simulink model "SimulinkOminidirectinalDrone_restored_from_autosave"  (R2025a)
settings: Solver=ode15s  StartTime=0.0  StopTime=10  RelTol=1e-4
values from neighbouring files (symbols this model uses):
  AUM = 3.057    [Parameter.m]
  g = -9.8    [Parameter.m]
  H = 0.05    [Parameter.m]
  L = 0.25    [Parameter.m]
  rho = 1.18195    [Parameter.m]
  W = diag([0.994, 0.003, 0.003, 0.994, 0.003, 0.003,            0.994, 0.003, 0.003, 0.994, 0.003, 0.003])    [Parameter.m]
libraries: slpidlib x10, matrix_library x8, robotcorelib x4, simulink x1, uavalgslib x1, aerolibobsolete x1
(part 1 of 2)
settings Model: Creator=Nguyen_Duc  LastModifiedBy=Nguyen_Duc
settings RTWCC: GPUComputeCapability=3.5

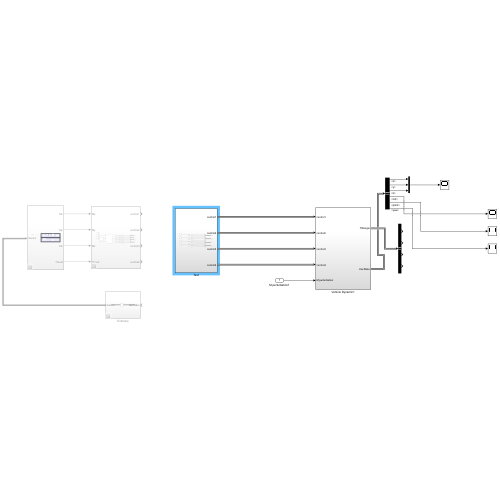
[thumbnail: Simulink's stored preview of the top-level diagram]
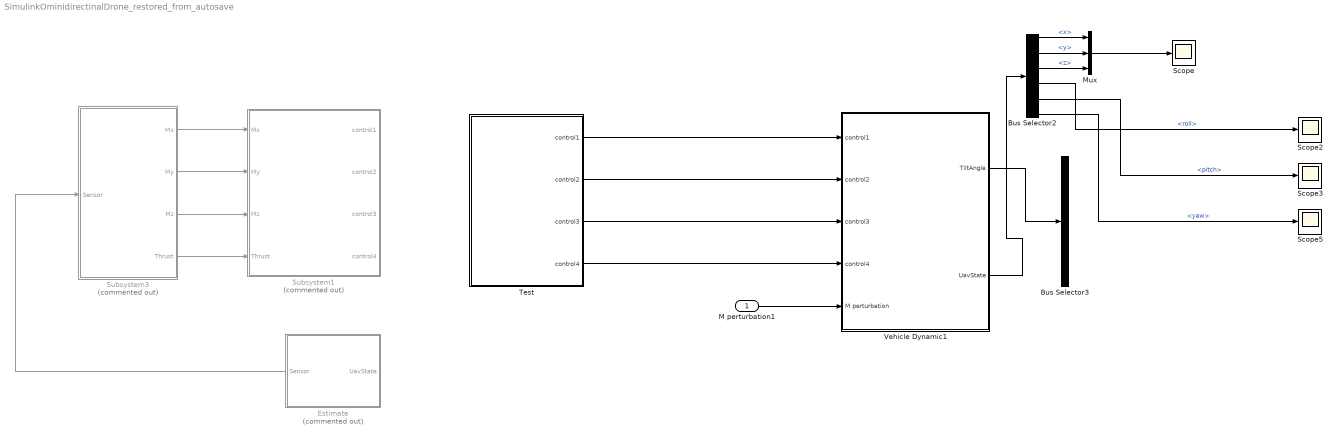
== system SimulinkOminidirectinalDrone_restored_from_autosave ==
  M perturbation1 : Inport
  Bus Selector2 : BusSelector  OutputSignals=x,y,z,roll,pitch,yaw
  Bus Selector3 : BusSelector  OutputSignals=signal1,signal2,signal3,signal4
  Estimate : Subsystem  Commented=on
  Mux : Mux  Inputs=3
  Scope{,2..3,5} (4 alike) : Scope
      Scope settings: ActiveDisplayYMinimum=-3203.8909963657634  ActiveDisplayYMaximum=3110.7651508209105
      Scope2 settings: ActiveDisplayYMinimum=-2.0964114847916129  ActiveDisplayYMaximum=2.211139771042796  DataLoggingVariableName=ScopeData2
      Scope3 settings: ActiveDisplayYMinimum=-3.8093227520417652  ActiveDisplayYMaximum=3.6702175311661223  DataLoggingVariableName=ScopeData3
      Scope5 settings: ActiveDisplayYMinimum=-9.534765072380404  ActiveDisplayYMaximum=7.24447859071625  DataLoggingVariableName=ScopeData5
  Subsystem1 : Subsystem  Commented=on
  Subsystem3 : Subsystem  Commented=on
  Test : Subsystem
  Vehicle Dynamic1 : Subsystem
  wires:
  Bus Selector2/1 -> Mux/1  "<x>"
  Subsystem3/3(Mz) -> Subsystem1/3(Mz)
  Subsystem3/1(Mx) -> Subsystem1/1(Mx)
  Bus Selector2/5 -> Scope3/1  "<pitch>"
  Subsystem3/2(My) -> Subsystem1/2(My)
  M perturbation1/1 -> Vehicle Dynamic1/5(M perturbation)
  Vehicle Dynamic1/1(TiltAngle) -> Bus Selector3/1
  Bus Selector2/6 -> Scope5/1  "<yaw>"
  Bus Selector2/3 -> Mux/3  "<z>"
  Subsystem3/4(Thrust) -> Subsystem1/4(Thrust)
  Bus Selector2/4 -> Scope2/1  "<roll>"
  Bus Selector2/2 -> Mux/2  "<y>"
  Vehicle Dynamic1/2(UavState) -> Bus Selector2/1
  Mux/1 -> Scope/1
  Estimate/1(Sensor) -> Subsystem3/1(Sensor)
  Test/1(control1) -> Vehicle Dynamic1/1(control1)
  Test/2(control2) -> Vehicle Dynamic1/2(control2)
  Test/3(control3) -> Vehicle Dynamic1/3(control3)
  Test/4(control4) -> Vehicle Dynamic1/4(control4)

== system SimulinkOminidirectinalDrone_restored_from_autosave/Estimate ==
  UavState : Inport
  Rate Transition : RateTransition  OutPortSampleTime=0.005
  Sensor : Outport
  wires:
  UavState/1 -> Rate Transition/1
  Rate Transition/1 -> Sensor/1

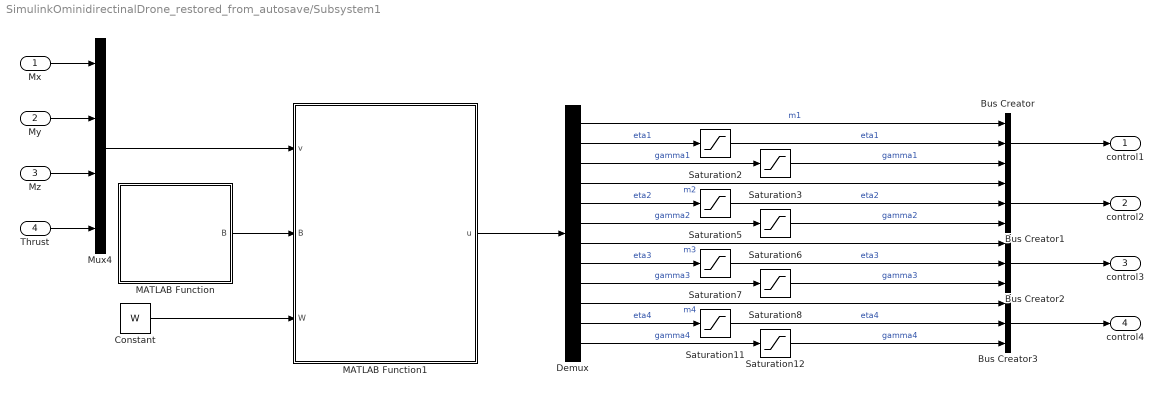
== system SimulinkOminidirectinalDrone_restored_from_autosave/Subsystem1 ==
  Mx : Inport
  My : Inport  Port=2
  Mz : Inport  Port=3
  Thrust : Inport  Port=4
  Bus Creator{,1..3} (4 alike) : BusCreator  Inputs=3
  Constant : Constant  Value=W
  Demux : Demux  Outputs=12
  MATLAB Function : MATLAB Function  TreatAsAtomicUnit=on
  MATLAB Function1 : MATLAB Function  TreatAsAtomicUnit=on
  Mux4 : Mux
  Saturation{2..3,5..8,11..12} (8 alike) : Saturate  UpperLimit=20*pi/180  LowerLimit=-20*pi/180
  control1 : Outport
  control2 : Outport  Port=2
  control3 : Outport  Port=3
  control4 : Outport  Port=4
  wires:
  MATLAB Function/1(B) -> MATLAB Function1/2(B)
  Mux4/1 -> MATLAB Function1/1(v)
  Demux/1 -> Bus Creator/1  "m1"
  Bus Creator/1 -> control1/1
  Demux/3 -> Saturation3/1  "gamma1"
  Demux/2 -> Saturation2/1  "eta1"
  Demux/4 -> Bus Creator1/1  "m2"
  Demux/5 -> Saturation5/1  "eta2"
  Demux/6 -> Saturation6/1  "gamma2"
  Demux/7 -> Bus Creator2/1  "m3"
  Demux/8 -> Saturation7/1  "eta3"
  Demux/9 -> Saturation8/1  "gamma3"
  Demux/10 -> Bus Creator3/1  "m4"
  Demux/11 -> Saturation11/1  "eta4"
  Demux/12 -> Saturation12/1  "gamma4"
  Bus Creator1/1 -> control2/1
  Bus Creator2/1 -> control3/1
  Bus Creator3/1 -> control4/1
  Mx/1 -> Mux4/1
  My/1 -> Mux4/2
  Mz/1 -> Mux4/3
  Thrust/1 -> Mux4/4
  Constant/1 -> MATLAB Function1/3(W)
  MATLAB Function1/1(u) -> Demux/1
  Saturation2/1 -> Bus Creator/2  "eta1"
  Saturation3/1 -> Bus Creator/3  "gamma1"
  Saturation5/1 -> Bus Creator1/2  "eta2"
  Saturation6/1 -> Bus Creator1/3  "gamma2"
  Saturation7/1 -> Bus Creator2/2  "eta3"
  Saturation8/1 -> Bus Creator2/3  "gamma3"
  Saturation11/1 -> Bus Creator3/2  "eta4"
  Saturation12/1 -> Bus Creator3/3  "gamma4"

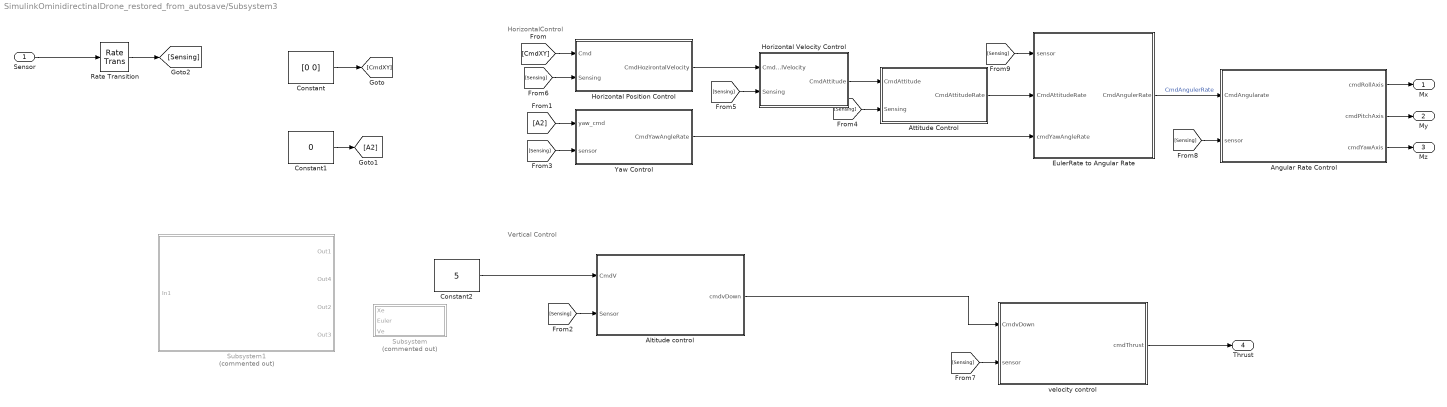
== system SimulinkOminidirectinalDrone_restored_from_autosave/Subsystem3 ==
  note: HorizontalControl
  note: Vertical Control
  Sensor : Inport
  Altitude control : Subsystem
  Angular Rate Control : Subsystem
  Attitude Control : Subsystem
  Constant : Constant  Value=[0 0]
  Constant1 : Constant  Value=0
  Constant2 : Constant  Value=5
  EulerRate to Angular Rate : Subsystem
  Horizontal Position Control : Subsystem
  Horizontal Velocity Control : Subsystem
  Rate Transition : RateTransition  OutPortSampleTime=0.005
  Subsystem : Subsystem  Commented=on
  Subsystem1 : Subsystem  Commented=on
  Yaw Control : Subsystem
  velocity control : Subsystem
  Mx : Outport
  My : Outport  Port=2
  Mz : Outport  Port=3
  Thrust : Outport  Port=4
  wires:
  Sensor/1 -> Rate Transition/1
  velocity control/1(cmdThrust) -> Thrust/1
  Altitude control/1(cmdvDown) -> velocity control/1(CmdvDown)
  EulerRate to Angular Rate/1(CmdAngulerRate) -> Angular Rate Control/1(CmdAngularate)  "CmdAngulerRate"
  Attitude Control/1(CmdAttitudeRate) -> EulerRate to Angular Rate/2(CmdAttitudeRate)
  Horizontal Velocity Control/1(CmdAttitude) -> Attitude Control/1(CmdAttitude)
  Horizontal Position Control/1(CmdHozirontalVelocity) -> Horizontal Velocity Control/1(CmdHozirontalVelocity)
  Yaw Control/1(CmdYawAngleRate) -> EulerRate to Angular Rate/3(cmdYawAngleRate)
  Angular Rate Control/1(cmdRollAxis) -> Mx/1
  Angular Rate Control/3(cmdYawAxis) -> Mz/1
  Angular Rate Control/2(cmdPitchAxis) -> My/1
  Constant/1 -> [CmdXY]
  [CmdXY] -> Horizontal Position Control/1(Cmd)
  Constant1/1 -> [A2]
  [A2] -> Yaw Control/1(yaw_cmd)
  Constant2/1 -> Altitude control/1(CmdV)
  Rate Transition/1 -> [Sensing]
  [Sensing] -> Altitude control/2(Sensor)
  [Sensing] -> Yaw Control/2(sensor)
  [Sensing] -> Attitude Control/2(Sensing)
  [Sensing] -> Horizontal Velocity Control/2(Sensing)
  [Sensing] -> Horizontal Position Control/2(Sensing)
  [Sensing] -> velocity control/2(sensor)
  [Sensing] -> Angular Rate Control/2(sensor)
  [Sensing] -> EulerRate to Angular Rate/1(sensor)

== system SimulinkOminidirectinalDrone_restored_from_autosave/Test ==
  Bus Creator{,1..3} (4 alike) : BusCreator  Inputs=3
  Constant : Constant  Value=2000
  Constant{1..2,4..5,7..8,10..11} (8 alike) : Constant
  Constant3 : Constant  Value=2000
  Constant6 : Constant  Value=1000
  Constant9 : Constant  Value=2000
  control1 : Outport
  control2 : Outport  Port=2
  control3 : Outport  Port=3
  control4 : Outport  Port=4
  wires:
  Constant1/1 -> Bus Creator/2  "eta1"
  Bus Creator1/1 -> control2/1
  Constant4/1 -> Bus Creator1/2  "eta2"
  Constant5/1 -> Bus Creator1/3  "gamma2"
  Bus Creator2/1 -> control3/1
  Constant3/1 -> Bus Creator1/1  "m2"
  Constant10/1 -> Bus Creator3/2  "eta4"
  Constant2/1 -> Bus Creator/3  "gamma1"
  Bus Creator/1 -> control1/1
  Constant7/1 -> Bus Creator2/2  "eta3"
  Constant11/1 -> Bus Creator3/3  "gamma4"
  Constant8/1 -> Bus Creator2/3  "gamma3"
  Bus Creator3/1 -> control4/1
  Constant6/1 -> Bus Creator2/1  "m3"
  Constant/1 -> Bus Creator/1  "m1"
  Constant9/1 -> Bus Creator3/1  "m4"

== system SimulinkOminidirectinalDrone_restored_from_autosave/Vehicle Dynamic1 ==
  control1 : Inport
  control2 : Inport  Port=2
  control3 : Inport  Port=3
  control4 : Inport  Port=4
  M perturbation : Inport  Port=5
  6DOF (Euler Angles) : aerolibobsolete/6DOF (Euler Angles)  units=Metric (MKS)  mtype=Fixed  rep=Euler Angles  xme_0=[0 0 0]  Vm_0=[0 0 0]  eul_0=[0 0 0]  pm_0=[0 0 0]  mass_0=AUM  mass_e=0.5  mass_f=2.0  inertia=[0.049827 0 0; 0 0.048993 0; 0 0 0.082777]  inertia_e=eye(3)  inertia_f=2*eye(3)  k_quat=1.0  vre_flag=on  abi_flag=off  aMode=0  xme_statename=''  Vm_statename=''  eul_statename=''  quat_statename=''  pm_statename=''  mass_statename=''
  Constant : Constant  Value=[0 0 g*AUM]'
  Matrix Multiply : Product  Multiplication=Matrix(*)
  Subsystem1 : Subsystem
  Sum : Sum  Inputs=++|
  Sum1 : Sum  Inputs=|++
  Uav : Subsystem
  actuator : Subsystem
  TiltAngle : Outport
  UavState : Outport  Port=2
  wires:
  control3/1 -> actuator/4(control3)
  M perturbation/1 -> Sum1/2
  Matrix Multiply/1 -> Sum/1
  control1/1 -> actuator/2(control1)
  control2/1 -> actuator/3(control2)
  control4/1 -> actuator/5(control4)
  Constant/1 -> Matrix Multiply/2
  6DOF (Euler Angles)/6 -> Uav/6(pqr), Subsystem1/1(omega)  "pqr"
  6DOF (Euler Angles)/5 -> Uav/5(vb), actuator/6(Vb)  "vb"
  6DOF (Euler Angles)/4 -> Uav/4(dcm), Matrix Multiply/1  "dcm"
  actuator/3(TiltAngle) -> TiltAngle/1
  Subsystem1/1(Rotation) -> actuator/1(rotation)
  Sum/1 -> 6DOF (Euler Angles)/1
  actuator/1(Forces) -> Sum/2
  actuator/2(Moments) -> Sum1/1
  Sum1/1 -> 6DOF (Euler Angles)/2
  6DOF (Euler Angles)/1 -> Uav/1(ve)  "ve"
  6DOF (Euler Angles)/2 -> Uav/2(xe)  "xe"
  6DOF (Euler Angles)/3 -> Uav/3(euler)  "euler"
  6DOF (Euler Angles)/7 -> Uav/7(angular acce)  "angular acce"
  6DOF (Euler Angles)/8 -> Uav/8(accel)  "accel"
  Uav/1(UavState) -> UavState/1

== system SimulinkOminidirectinalDrone_restored_from_autosave/Subsystem3/Altitude control ==
  CmdV : Inport
  In Bus Element1 : Inport  Port=2  PortName=Sensor  Element=z
  Discrete PID Controller : slpidlib/PID Controller  Controller=PD  Form=Parallel  TimeDomain=Discrete-time  UseExternalTs=off  SampleTime=0.005  IntegratorMethod=Forward Euler  FilterMethod=Forward Euler  ControllerParametersSource=internal  P=100  I=1  UseKiTs=off  D=1000  UseExternalDerivativeSource=off  N=100  UseFilter=on  TunerSelectOption=Transfer Function Based (PID Tuner App)  InitialConditionSource=external  InitialConditionForIntegrator=0  InitialConditionForFilter=0  DifferentiatorICPrevScaledInput=0  ExternalReset=none  TrackingMode=off  Kt=1  LimitOutput=on  SatLimitsSource=internal  UpperSaturationLimit=inf  LowerSaturationLimit=-inf  LinearizeAsGain=off  AntiWindupMode=none  Kb=1  LimitIntegrator=off  UpperIntegratorSaturationLimit=inf  LowerIntegratorSaturationLimit=-inf  POutMin=[]  POutMax=[]  IOutMin=[]  IOutMax=[]  DOutMin=[]  DOutMax=[]  NOutMin=[]  NOutMax=[]  SumOutMin=[]  SumOutMax=[]  SaturationOutMin=[]  SaturationOutMax=[]  PParamMin=[]  PParamMax=[]  IParamMin=[]  IParamMax=[]  DParamMin=[]  DParamMax=[]  NParamMin=[]  NParamMax=[]  KbParamMin=[]  KbParamMax=[]  KtParamMin=[]  KtParamMax=[]  KbOutMin=[]  KbOutMax=[]  KtOutMin=[]  KtOutMax=[]  IntegratorOutMin=[]  IntegratorOutMax=[]  FilterOutMin=[]  FilterOutMax=[]  SumI1OutMin=[]  SumI1OutMax=[]  SumI2OutMin=[]  SumI2OutMax=[]  SumI3OutMin=[]  SumI3OutMax=[]  SumI4OutMin=[]  SumI4OutMax=[]  SumDOutMin=[]  SumDOutMax=[]  DifferentiatorOutMin=[]  DifferentiatorOutMax=[]  FilterDiffOutCoefMin=[]  FilterDiffOutCoefMax=[]  ReciprocalOutMin=[]  ReciprocalOutMax=[]  SumDenOutMin=[]  SumDenOutMax=[]  SumNumOutMin=[]  SumNumOutMax=[]  DivideOutMin=[]  DivideOutMax=[]  UdiffTsProdOutMin=[]  UdiffTsProdOutMax=[]  NTsProdOutMin=[]  NTsProdOutMax=[]  UintegralTsProdOutMin=[]  UintegralTsProdOutMax=[]  UngainTsProdOutMin=[]  UngainTsProdOutMax=[]  ClampingZeroOutDataTypeStr=Inherit: Inherit via back propagation  ClampingZeroOutMin=[]  ClampingZeroOutMax=[]  FilterDenConstantOutDataTypeStr=Inherit: Inherit via back propagation  FilterDenConstantOutMin=[]  FilterDenConstantOutMax=[]  PCopyOutDataTypeStr=Inherit: Inherit via back propagation  PCopyOutMin=[]  PCopyOutMax=[]  NCopyOutDataTypeStr=Inherit: Inherit via back propagation  NCopyOutMin=[]  NCopyOutMax=[]  IntegratorContinuousStateAttributes=''  IntegratorStateMustResolveToSignalObject=off  IntegratorRTWStateStorageClass=Auto  FilterContinuousStateAttributes=''  FilterStateMustResolveToSignalObject=off  FilterRTWStateStorageClass=Auto  ParallelPVariant=InternalParameters  IdealPVariant=Disabled  IVariant=Disabled  DVariant=InternalParameters  IntegratorVariant=Disabled  SatVariant=Enabled  AWVariant=Disabled  PCopyVariant=Disabled  TRVariant=Disabled  FdbkBlocksVariant=Forward  IdealPFdbkVariant=Disabled  SatFdbkVariant=Disabled  DerivativeFilterVariant=ForwardEulerFilter  NVariant=InternalParameters  NCopyVariant=Disabled  FilterICVariant=ExternalICs  IntegratorICVariant=Disabled  ExternalResetVariant=Disabled  TRSumVariant=Passthrough  SumFdbkVariant=Disabled  SumVariant=Sum_PD  TsampFilterVariant=InternalTs  TsampNgainVariant=Passthrough  TsampIntegralVariant=Disabled_SignalSpec  ExternalSaturationOutDataTypeStr=Inherit: Same as second input  DerivativeSourceVariant=ErrorSignal  PreIntVariant=InternalPreInt
      settings: LibrarySourceBlock=simulink/Discrete/Discrete PID Controller
  Gain : Gain  Gain=-2
  Sum : Sum  Inputs=|+-
  cmdvDown : Outport
  wires:
  Sum/1 -> Discrete PID Controller/1
  In Bus Element1/1 -> Sum/2
  CmdV/1 -> Gain/1
  Discrete PID Controller/1 -> cmdvDown/1  "cmdvDown"
  Gain/1 -> Sum/1

== system SimulinkOminidirectinalDrone_restored_from_autosave/Subsystem3/Angular Rate Control ==
  In Bus Element : Inport  PortName=CmdAngularate  Element=wx
  In Bus Element1 : Inport  PortName=CmdAngularate  Element=wy
  In Bus Element4 : Inport  PortName=CmdAngularate  Element=wz
  In Bus Element2 : Inport  Port=2  PortName=sensor  Element=wy
  In Bus Element3 : Inport  Port=2  PortName=sensor  Element=wx
  In Bus Element5 : Inport  Port=2  PortName=sensor  Element=wz
  Demux : Demux  Outputs=2
  Discrete PID Controller : slpidlib/PID Controller  Controller=PID  Form=Parallel  TimeDomain=Discrete-time  UseExternalTs=off  SampleTime=-1  IntegratorMethod=Forward Euler  FilterMethod=Forward Euler  ControllerParametersSource=internal  P=1  I=0  UseKiTs=off  D=0  UseExternalDerivativeSource=off  N=100  UseFilter=on  TunerSelectOption=Transfer Function Based (PID Tuner App)  InitialConditionSource=internal  InitialConditionForIntegrator=0  InitialConditionForFilter=0  DifferentiatorICPrevScaledInput=0  ExternalReset=none  TrackingMode=off  Kt=1  LimitOutput=off  SatLimitsSource=internal  UpperSaturationLimit=inf  LowerSaturationLimit=-inf  LinearizeAsGain=off  AntiWindupMode=none  Kb=1  LimitIntegrator=off  UpperIntegratorSaturationLimit=inf  LowerIntegratorSaturationLimit=-inf  POutMin=[]  POutMax=[]  IOutMin=[]  IOutMax=[]  DOutMin=[]  DOutMax=[]  NOutMin=[]  NOutMax=[]  SumOutMin=[]  SumOutMax=[]  SaturationOutMin=[]  SaturationOutMax=[]  PParamMin=[]  PParamMax=[]  IParamMin=[]  IParamMax=[]  DParamMin=[]  DParamMax=[]  NParamMin=[]  NParamMax=[]  KbParamMin=[]  KbParamMax=[]  KtParamMin=[]  KtParamMax=[]  KbOutMin=[]  KbOutMax=[]  KtOutMin=[]  KtOutMax=[]  IntegratorOutMin=[]  IntegratorOutMax=[]  FilterOutMin=[]  FilterOutMax=[]  SumI1OutMin=[]  SumI1OutMax=[]  SumI2OutMin=[]  SumI2OutMax=[]  SumI3OutMin=[]  SumI3OutMax=[]  SumI4OutMin=[]  SumI4OutMax=[]  SumDOutMin=[]  SumDOutMax=[]  DifferentiatorOutMin=[]  DifferentiatorOutMax=[]  FilterDiffOutCoefMin=[]  FilterDiffOutCoefMax=[]  ReciprocalOutMin=[]  ReciprocalOutMax=[]  SumDenOutMin=[]  SumDenOutMax=[]  SumNumOutMin=[]  SumNumOutMax=[]  DivideOutMin=[]  DivideOutMax=[]  UdiffTsProdOutMin=[]  UdiffTsProdOutMax=[]  NTsProdOutMin=[]  NTsProdOutMax=[]  UintegralTsProdOutMin=[]  UintegralTsProdOutMax=[]  UngainTsProdOutMin=[]  UngainTsProdOutMax=[]  ClampingZeroOutDataTypeStr=Inherit: Inherit via back propagation  ClampingZeroOutMin=[]  ClampingZeroOutMax=[]  FilterDenConstantOutDataTypeStr=Inherit: Inherit via back propagation  FilterDenConstantOutMin=[]  FilterDenConstantOutMax=[]  PCopyOutDataTypeStr=Inherit: Inherit via back propagation  PCopyOutMin=[]  PCopyOutMax=[]  NCopyOutDataTypeStr=Inherit: Inherit via back propagation  NCopyOutMin=[]  NCopyOutMax=[]  IntegratorContinuousStateAttributes=''  IntegratorStateMustResolveToSignalObject=off  IntegratorRTWStateStorageClass=Auto  FilterContinuousStateAttributes=''  FilterStateMustResolveToSignalObject=off  FilterRTWStateStorageClass=Auto  ParallelPVariant=InternalParameters  IdealPVariant=Disabled  IVariant=InternalParameters  DVariant=InternalParameters  IntegratorVariant=Discrete  SatVariant=Disabled  AWVariant=Passthrough  PCopyVariant=Disabled  TRVariant=Disabled  FdbkBlocksVariant=Forward  IdealPFdbkVariant=Disabled  SatFdbkVariant=Disabled  DerivativeFilterVariant=ForwardEulerFilter  NVariant=InternalParameters  NCopyVariant=Disabled  FilterICVariant=InternalICsFilter  IntegratorICVariant=InternalICs  ExternalResetVariant=Disabled  TRSumVariant=Passthrough  SumFdbkVariant=Disabled  SumVariant=Sum_PID  TsampFilterVariant=InternalTs  TsampNgainVariant=Passthrough  TsampIntegralVariant=Disabled_SignalSpec  ExternalSaturationOutDataTypeStr=Inherit: Same as second input  DerivativeSourceVariant=ErrorSignal  PreIntVariant=InternalPreInt
      settings: LibrarySourceBlock=simulink/Discrete/Discrete PID Controller
  Discrete PID Controller1 : slpidlib/PID Controller  Controller=PID  Form=Parallel  TimeDomain=Discrete-time  UseExternalTs=off  SampleTime=-1  IntegratorMethod=Forward Euler  FilterMethod=Forward Euler  ControllerParametersSource=internal  P=1  I=0  UseKiTs=off  D=0  UseExternalDerivativeSource=off  N=100  UseFilter=on  TunerSelectOption=Transfer Function Based (PID Tuner App)  InitialConditionSource=internal  InitialConditionForIntegrator=0  InitialConditionForFilter=0  DifferentiatorICPrevScaledInput=0  ExternalReset=none  TrackingMode=off  Kt=1  LimitOutput=off  SatLimitsSource=internal  UpperSaturationLimit=inf  LowerSaturationLimit=-inf  LinearizeAsGain=off  AntiWindupMode=none  Kb=1  LimitIntegrator=off  UpperIntegratorSaturationLimit=inf  LowerIntegratorSaturationLimit=-inf  POutMin=[]  POutMax=[]  IOutMin=[]  IOutMax=[]  DOutMin=[]  DOutMax=[]  NOutMin=[]  NOutMax=[]  SumOutMin=[]  SumOutMax=[]  SaturationOutMin=[]  SaturationOutMax=[]  PParamMin=[]  PParamMax=[]  IParamMin=[]  IParamMax=[]  DParamMin=[]  DParamMax=[]  NParamMin=[]  NParamMax=[]  KbParamMin=[]  KbParamMax=[]  KtParamMin=[]  KtParamMax=[]  KbOutMin=[]  KbOutMax=[]  KtOutMin=[]  KtOutMax=[]  IntegratorOutMin=[]  IntegratorOutMax=[]  FilterOutMin=[]  FilterOutMax=[]  SumI1OutMin=[]  SumI1OutMax=[]  SumI2OutMin=[]  SumI2OutMax=[]  SumI3OutMin=[]  SumI3OutMax=[]  SumI4OutMin=[]  SumI4OutMax=[]  SumDOutMin=[]  SumDOutMax=[]  DifferentiatorOutMin=[]  DifferentiatorOutMax=[]  FilterDiffOutCoefMin=[]  FilterDiffOutCoefMax=[]  ReciprocalOutMin=[]  ReciprocalOutMax=[]  SumDenOutMin=[]  SumDenOutMax=[]  SumNumOutMin=[]  SumNumOutMax=[]  DivideOutMin=[]  DivideOutMax=[]  UdiffTsProdOutMin=[]  UdiffTsProdOutMax=[]  NTsProdOutMin=[]  NTsProdOutMax=[]  UintegralTsProdOutMin=[]  UintegralTsProdOutMax=[]  UngainTsProdOutMin=[]  UngainTsProdOutMax=[]  ClampingZeroOutDataTypeStr=Inherit: Inherit via back propagation  ClampingZeroOutMin=[]  ClampingZeroOutMax=[]  FilterDenConstantOutDataTypeStr=Inherit: Inherit via back propagation  FilterDenConstantOutMin=[]  FilterDenConstantOutMax=[]  PCopyOutDataTypeStr=Inherit: Inherit via back propagation  PCopyOutMin=[]  PCopyOutMax=[]  NCopyOutDataTypeStr=Inherit: Inherit via back propagation  NCopyOutMin=[]  NCopyOutMax=[]  IntegratorContinuousStateAttributes=''  IntegratorStateMustResolveToSignalObject=off  IntegratorRTWStateStorageClass=Auto  FilterContinuousStateAttributes=''  FilterStateMustResolveToSignalObject=off  FilterRTWStateStorageClass=Auto  ParallelPVariant=InternalParameters  IdealPVariant=Disabled  IVariant=InternalParameters  DVariant=InternalParameters  IntegratorVariant=Discrete  SatVariant=Disabled  AWVariant=Passthrough  PCopyVariant=Disabled  TRVariant=Disabled  FdbkBlocksVariant=Forward  IdealPFdbkVariant=Disabled  SatFdbkVariant=Disabled  DerivativeFilterVariant=ForwardEulerFilter  NVariant=InternalParameters  NCopyVariant=Disabled  FilterICVariant=InternalICsFilter  IntegratorICVariant=InternalICs  ExternalResetVariant=Disabled  TRSumVariant=Passthrough  SumFdbkVariant=Disabled  SumVariant=Sum_PID  TsampFilterVariant=InternalTs  TsampNgainVariant=Passthrough  TsampIntegralVariant=Disabled_SignalSpec  ExternalSaturationOutDataTypeStr=Inherit: Same as second input  DerivativeSourceVariant=ErrorSignal  PreIntVariant=InternalPreInt
      settings: LibrarySourceBlock=simulink/Discrete/Discrete PID Controller
  Gain : Gain  Gain=20
  Gain1 : Gain  Gain=100
  Mux : Mux  Inputs=2
  Mux1 : Mux  Inputs=2
  Sum : Sum  Inputs=|+-
  Sum1 : Sum  Inputs=|+-
  cmdRollAxis : Outport
  cmdPitchAxis : Outport  Port=2
  cmdYawAxis : Outport  Port=3
  wires:
  In Bus Element/1 -> Mux/1
  In Bus Element1/1 -> Mux/2
  In Bus Element3/1 -> Mux1/1
  In Bus Element2/1 -> Mux1/2
  Mux/1 -> Sum/1
  Mux1/1 -> Sum/2
  Sum/1 -> Discrete PID Controller/1
  Discrete PID Controller/1 -> Gain/1
  Gain/1 -> Demux/1
  Demux/2 -> cmdPitchAxis/1
  Demux/1 -> cmdRollAxis/1
  In Bus Element4/1 -> Sum1/1
  In Bus Element5/1 -> Sum1/2
  Sum1/1 -> Discrete PID Controller1/1
  Discrete PID Controller1/1 -> Gain1/1
  Gain1/1 -> cmdYawAxis/1

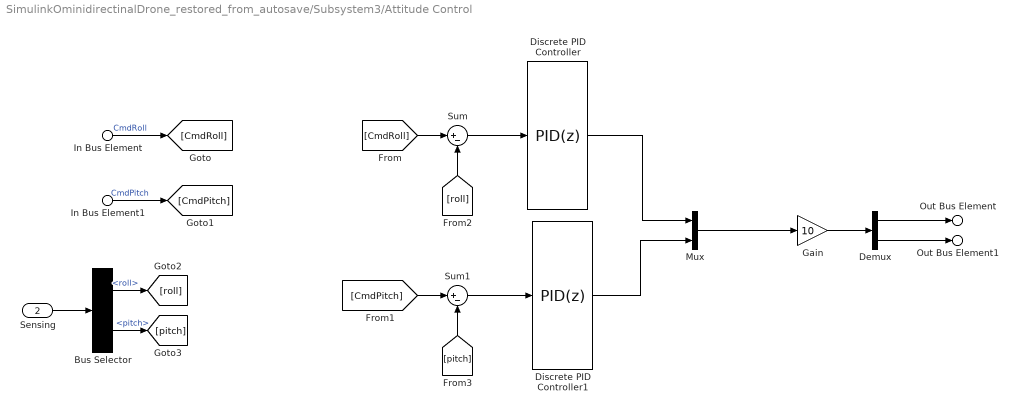
== system SimulinkOminidirectinalDrone_restored_from_autosave/Subsystem3/Attitude Control ==
  In Bus Element : Inport  PortName=CmdAttitude  Element=roll
  In Bus Element1 : Inport  PortName=CmdAttitude  Element=pitch
  Sensing : Inport  Port=2
  Bus Selector : BusSelector  OutputSignals=roll,pitch
  Demux : Demux  Outputs=2
  Discrete PID Controller : slpidlib/PID Controller  Controller=PID  Form=Parallel  TimeDomain=Discrete-time  UseExternalTs=off  SampleTime=-1  IntegratorMethod=Forward Euler  FilterMethod=Forward Euler  ControllerParametersSource=internal  P=1  I=0  UseKiTs=off  D=0  UseExternalDerivativeSource=off  N=100  UseFilter=on  TunerSelectOption=Transfer Function Based (PID Tuner App)  InitialConditionSource=internal  InitialConditionForIntegrator=0  InitialConditionForFilter=0  DifferentiatorICPrevScaledInput=0  ExternalReset=none  TrackingMode=off  Kt=1  LimitOutput=off  SatLimitsSource=internal  UpperSaturationLimit=inf  LowerSaturationLimit=-inf  LinearizeAsGain=off  AntiWindupMode=none  Kb=1  LimitIntegrator=off  UpperIntegratorSaturationLimit=inf  LowerIntegratorSaturationLimit=-inf  POutMin=[]  POutMax=[]  IOutMin=[]  IOutMax=[]  DOutMin=[]  DOutMax=[]  NOutMin=[]  NOutMax=[]  SumOutMin=[]  SumOutMax=[]  SaturationOutMin=[]  SaturationOutMax=[]  PParamMin=[]  PParamMax=[]  IParamMin=[]  IParamMax=[]  DParamMin=[]  DParamMax=[]  NParamMin=[]  NParamMax=[]  KbParamMin=[]  KbParamMax=[]  KtParamMin=[]  KtParamMax=[]  KbOutMin=[]  KbOutMax=[]  KtOutMin=[]  KtOutMax=[]  IntegratorOutMin=[]  IntegratorOutMax=[]  FilterOutMin=[]  FilterOutMax=[]  SumI1OutMin=[]  SumI1OutMax=[]  SumI2OutMin=[]  SumI2OutMax=[]  SumI3OutMin=[]  SumI3OutMax=[]  SumI4OutMin=[]  SumI4OutMax=[]  SumDOutMin=[]  SumDOutMax=[]  DifferentiatorOutMin=[]  DifferentiatorOutMax=[]  FilterDiffOutCoefMin=[]  FilterDiffOutCoefMax=[]  ReciprocalOutMin=[]  ReciprocalOutMax=[]  SumDenOutMin=[]  SumDenOutMax=[]  SumNumOutMin=[]  SumNumOutMax=[]  DivideOutMin=[]  DivideOutMax=[]  UdiffTsProdOutMin=[]  UdiffTsProdOutMax=[]  NTsProdOutMin=[]  NTsProdOutMax=[]  UintegralTsProdOutMin=[]  UintegralTsProdOutMax=[]  UngainTsProdOutMin=[]  UngainTsProdOutMax=[]  ClampingZeroOutDataTypeStr=Inherit: Inherit via back propagation  ClampingZeroOutMin=[]  ClampingZeroOutMax=[]  FilterDenConstantOutDataTypeStr=Inherit: Inherit via back propagation  FilterDenConstantOutMin=[]  FilterDenConstantOutMax=[]  PCopyOutDataTypeStr=Inherit: Inherit via back propagation  PCopyOutMin=[]  PCopyOutMax=[]  NCopyOutDataTypeStr=Inherit: Inherit via back propagation  NCopyOutMin=[]  NCopyOutMax=[]  IntegratorContinuousStateAttributes=''  IntegratorStateMustResolveToSignalObject=off  IntegratorRTWStateStorageClass=Auto  FilterContinuousStateAttributes=''  FilterStateMustResolveToSignalObject=off  FilterRTWStateStorageClass=Auto  ParallelPVariant=InternalParameters  IdealPVariant=Disabled  IVariant=InternalParameters  DVariant=InternalParameters  IntegratorVariant=Discrete  SatVariant=Disabled  AWVariant=Passthrough  PCopyVariant=Disabled  TRVariant=Disabled  FdbkBlocksVariant=Forward  IdealPFdbkVariant=Disabled  SatFdbkVariant=Disabled  DerivativeFilterVariant=ForwardEulerFilter  NVariant=InternalParameters  NCopyVariant=Disabled  FilterICVariant=InternalICsFilter  IntegratorICVariant=InternalICs  ExternalResetVariant=Disabled  TRSumVariant=Passthrough  SumFdbkVariant=Disabled  SumVariant=Sum_PID  TsampFilterVariant=InternalTs  TsampNgainVariant=Passthrough  TsampIntegralVariant=Disabled_SignalSpec  ExternalSaturationOutDataTypeStr=Inherit: Same as second input  DerivativeSourceVariant=ErrorSignal  PreIntVariant=InternalPreInt
      settings: LibrarySourceBlock=simulink/Discrete/Discrete PID Controller
  Discrete PID Controller1 : slpidlib/PID Controller  Controller=PID  Form=Parallel  TimeDomain=Discrete-time  UseExternalTs=off  SampleTime=-1  IntegratorMethod=Forward Euler  FilterMethod=Forward Euler  ControllerParametersSource=internal  P=1  I=0  UseKiTs=off  D=0  UseExternalDerivativeSource=off  N=100  UseFilter=on  TunerSelectOption=Transfer Function Based (PID Tuner App)  InitialConditionSource=internal  InitialConditionForIntegrator=0  InitialConditionForFilter=0  DifferentiatorICPrevScaledInput=0  ExternalReset=none  TrackingMode=off  Kt=1  LimitOutput=off  SatLimitsSource=internal  UpperSaturationLimit=inf  LowerSaturationLimit=-inf  LinearizeAsGain=off  AntiWindupMode=none  Kb=1  LimitIntegrator=off  UpperIntegratorSaturationLimit=inf  LowerIntegratorSaturationLimit=-inf  POutMin=[]  POutMax=[]  IOutMin=[]  IOutMax=[]  DOutMin=[]  DOutMax=[]  NOutMin=[]  NOutMax=[]  SumOutMin=[]  SumOutMax=[]  SaturationOutMin=[]  SaturationOutMax=[]  PParamMin=[]  PParamMax=[]  IParamMin=[]  IParamMax=[]  DParamMin=[]  DParamMax=[]  NParamMin=[]  NParamMax=[]  KbParamMin=[]  KbParamMax=[]  KtParamMin=[]  KtParamMax=[]  KbOutMin=[]  KbOutMax=[]  KtOutMin=[]  KtOutMax=[]  IntegratorOutMin=[]  IntegratorOutMax=[]  FilterOutMin=[]  FilterOutMax=[]  SumI1OutMin=[]  SumI1OutMax=[]  SumI2OutMin=[]  SumI2OutMax=[]  SumI3OutMin=[]  SumI3OutMax=[]  SumI4OutMin=[]  SumI4OutMax=[]  SumDOutMin=[]  SumDOutMax=[]  DifferentiatorOutMin=[]  DifferentiatorOutMax=[]  FilterDiffOutCoefMin=[]  FilterDiffOutCoefMax=[]  ReciprocalOutMin=[]  ReciprocalOutMax=[]  SumDenOutMin=[]  SumDenOutMax=[]  SumNumOutMin=[]  SumNumOutMax=[]  DivideOutMin=[]  DivideOutMax=[]  UdiffTsProdOutMin=[]  UdiffTsProdOutMax=[]  NTsProdOutMin=[]  NTsProdOutMax=[]  UintegralTsProdOutMin=[]  UintegralTsProdOutMax=[]  UngainTsProdOutMin=[]  UngainTsProdOutMax=[]  ClampingZeroOutDataTypeStr=Inherit: Inherit via back propagation  ClampingZeroOutMin=[]  ClampingZeroOutMax=[]  FilterDenConstantOutDataTypeStr=Inherit: Inherit via back propagation  FilterDenConstantOutMin=[]  FilterDenConstantOutMax=[]  PCopyOutDataTypeStr=Inherit: Inherit via back propagation  PCopyOutMin=[]  PCopyOutMax=[]  NCopyOutDataTypeStr=Inherit: Inherit via back propagation  NCopyOutMin=[]  NCopyOutMax=[]  IntegratorContinuousStateAttributes=''  IntegratorStateMustResolveToSignalObject=off  IntegratorRTWStateStorageClass=Auto  FilterContinuousStateAttributes=''  FilterStateMustResolveToSignalObject=off  FilterRTWStateStorageClass=Auto  ParallelPVariant=InternalParameters  IdealPVariant=Disabled  IVariant=InternalParameters  DVariant=InternalParameters  IntegratorVariant=Discrete  SatVariant=Disabled  AWVariant=Passthrough  PCopyVariant=Disabled  TRVariant=Disabled  FdbkBlocksVariant=Forward  IdealPFdbkVariant=Disabled  SatFdbkVariant=Disabled  DerivativeFilterVariant=ForwardEulerFilter  NVariant=InternalParameters  NCopyVariant=Disabled  FilterICVariant=InternalICsFilter  IntegratorICVariant=InternalICs  ExternalResetVariant=Disabled  TRSumVariant=Passthrough  SumFdbkVariant=Disabled  SumVariant=Sum_PID  TsampFilterVariant=InternalTs  TsampNgainVariant=Passthrough  TsampIntegralVariant=Disabled_SignalSpec  ExternalSaturationOutDataTypeStr=Inherit: Same as second input  DerivativeSourceVariant=ErrorSignal  PreIntVariant=InternalPreInt
      settings: LibrarySourceBlock=simulink/Discrete/Discrete PID Controller
  Gain : Gain  Gain=10
  Mux : Mux  Inputs=2
  Sum : Sum  Inputs=|+-
  Sum1 : Sum  Inputs=|+-
  Out Bus Element : Outport  PortName=CmdAttitudeRate  Element=roll
  Out Bus Element1 : Outport  PortName=CmdAttitudeRate  Element=pitch
  wires:
  Sum/1 -> Discrete PID Controller/1
  Gain/1 -> Demux/1
  Demux/1 -> Out Bus Element/1
  Demux/2 -> Out Bus Element1/1
  Sensing/1 -> Bus Selector/1
  Sum1/1 -> Discrete PID Controller1/1
  In Bus Element1/1 -> [CmdPitch]  "CmdPitch"
  [CmdPitch] -> Sum1/1
  Bus Selector/1 -> [roll]  "<roll>"
  [roll] -> Sum/2
  Bus Selector/2 -> [pitch]  "<pitch>"
  [pitch] -> Sum1/2
  Discrete PID Controller/1 -> Mux/1
  Discrete PID Controller1/1 -> Mux/2
  Mux/1 -> Gain/1
  In Bus Element/1 -> [CmdRoll]  "CmdRoll"
  [CmdRoll] -> Sum/1

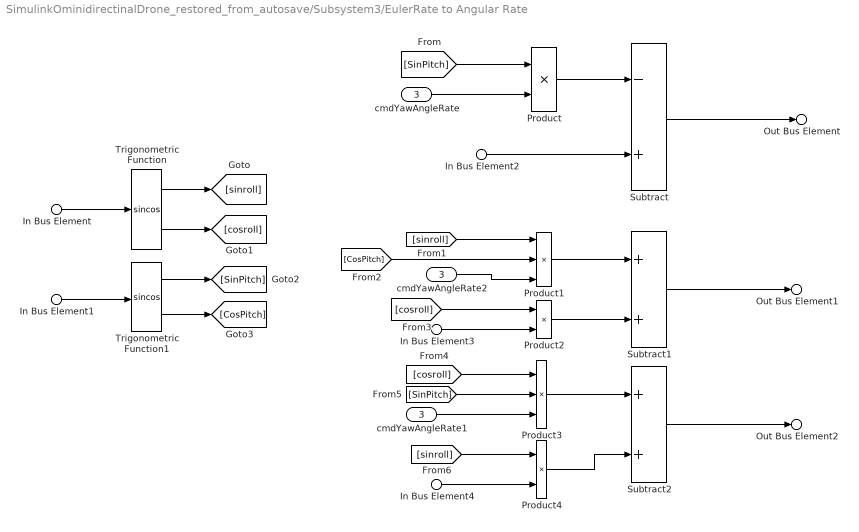
== system SimulinkOminidirectinalDrone_restored_from_autosave/Subsystem3/EulerRate to Angular Rate ==
  In Bus Element : Inport  PortName=sensor  Element=roll
  In Bus Element1 : Inport  PortName=sensor  Element=pitch
  In Bus Element2 : Inport  Port=2  PortName=CmdAttitudeRate  Element=roll
  In Bus Element4 : Inport  Port=2  PortName=CmdAttitudeRate  Element=pitch
  In Bus Element3 : Inport  Port=2  PortName=CmdAttitudeRate  Element=pitch
  cmdYawAngleRate : Inport  Port=3
  Product : Product
  Product1 : Product  Inputs=3
  Product2 : Product
  Product3 : Product  Inputs=3
  Product4 : Product
  Subtract : Sum  Inputs=-+
  Subtract1 : Sum
  Subtract2 : Sum
  Trigonometric Function : Trigonometry  Operator=sincos
  Trigonometric Function1 : Trigonometry  Operator=sincos
  cmdYawAngleRate1 : InportShadow  Port=3
  cmdYawAngleRate2 : InportShadow  Port=3
  Out Bus Element : Outport  PortName=CmdAngulerRate  Element=wx
  Out Bus Element1 : Outport  PortName=CmdAngulerRate  Element=wy
  Out Bus Element2 : Outport  PortName=CmdAngulerRate  Element=wz
  wires:
  In Bus Element/1 -> Trigonometric Function/1
  In Bus Element1/1 -> Trigonometric Function1/1
  Trigonometric Function/1 -> [sinroll]
  Trigonometric Function/2 -> [cosroll]
  Trigonometric Function1/1 -> [SinPitch]
  Trigonometric Function1/2 -> [CosPitch]
  [SinPitch] -> Product/1
  Product/1 -> Subtract/1
  In Bus Element2/1 -> Subtract/2
  [sinroll] -> Product1/1
  [CosPitch] -> Product1/2
  Product1/1 -> Subtract1/1
  [cosroll] -> Product2/1
  In Bus Element3/1 -> Product2/2
  Product3/1 -> Subtract2/1
  cmdYawAngleRate/1 -> Product/2
  [SinPitch] -> Product3/2
  [cosroll] -> Product3/1
  Product2/1 -> Subtract1/2
  [sinroll] -> Product4/1
  In Bus Element4/1 -> Product4/2
  cmdYawAngleRate2/1 -> Product1/3
  cmdYawAngleRate1/1 -> Product3/3
  Product4/1 -> Subtract2/2
  Subtract/1 -> Out Bus Element/1
  Subtract2/1 -> Out Bus Element2/1
  Subtract1/1 -> Out Bus Element1/1

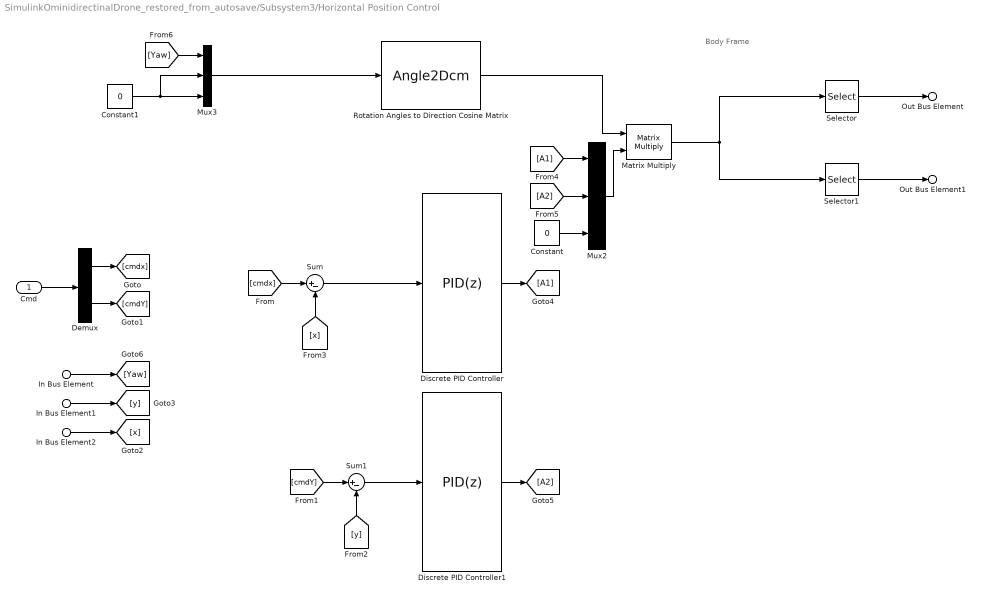
== system SimulinkOminidirectinalDrone_restored_from_autosave/Subsystem3/Horizontal Position Control ==
  note: Body Frame
  Cmd : Inport
  In Bus Element : Inport  Port=2  PortName=Sensing  Element=yaw
  In Bus Element1 : Inport  Port=2  PortName=Sensing  Element=y
  In Bus Element2 : Inport  Port=2  PortName=Sensing  Element=x
  Constant : Constant  Value=0
  Constant1 : Constant  Value=0
  Demux : Demux  Outputs=2
  Discrete PID Controller : slpidlib/PID Controller  Controller=PID  Form=Parallel  TimeDomain=Discrete-time  UseExternalTs=off  SampleTime=-1  IntegratorMethod=Forward Euler  FilterMethod=Forward Euler  ControllerParametersSource=internal  P=1  I=0  UseKiTs=off  D=0  UseExternalDerivativeSource=off  N=100  UseFilter=on  TunerSelectOption=Transfer Function Based (PID Tuner App)  InitialConditionSource=internal  InitialConditionForIntegrator=0  InitialConditionForFilter=0  DifferentiatorICPrevScaledInput=0  ExternalReset=none  TrackingMode=off  Kt=1  LimitOutput=off  SatLimitsSource=internal  UpperSaturationLimit=inf  LowerSaturationLimit=-inf  LinearizeAsGain=off  AntiWindupMode=none  Kb=1  LimitIntegrator=off  UpperIntegratorSaturationLimit=inf  LowerIntegratorSaturationLimit=-inf  POutMin=[]  POutMax=[]  IOutMin=[]  IOutMax=[]  DOutMin=[]  DOutMax=[]  NOutMin=[]  NOutMax=[]  SumOutMin=[]  SumOutMax=[]  SaturationOutMin=[]  SaturationOutMax=[]  PParamMin=[]  PParamMax=[]  IParamMin=[]  IParamMax=[]  DParamMin=[]  DParamMax=[]  NParamMin=[]  NParamMax=[]  KbParamMin=[]  KbParamMax=[]  KtParamMin=[]  KtParamMax=[]  KbOutMin=[]  KbOutMax=[]  KtOutMin=[]  KtOutMax=[]  IntegratorOutMin=[]  IntegratorOutMax=[]  FilterOutMin=[]  FilterOutMax=[]  SumI1OutMin=[]  SumI1OutMax=[]  SumI2OutMin=[]  SumI2OutMax=[]  SumI3OutMin=[]  SumI3OutMax=[]  SumI4OutMin=[]  SumI4OutMax=[]  SumDOutMin=[]  SumDOutMax=[]  DifferentiatorOutMin=[]  DifferentiatorOutMax=[]  FilterDiffOutCoefMin=[]  FilterDiffOutCoefMax=[]  ReciprocalOutMin=[]  ReciprocalOutMax=[]  SumDenOutMin=[]  SumDenOutMax=[]  SumNumOutMin=[]  SumNumOutMax=[]  DivideOutMin=[]  DivideOutMax=[]  UdiffTsProdOutMin=[]  UdiffTsProdOutMax=[]  NTsProdOutMin=[]  NTsProdOutMax=[]  UintegralTsProdOutMin=[]  UintegralTsProdOutMax=[]  UngainTsProdOutMin=[]  UngainTsProdOutMax=[]  ClampingZeroOutDataTypeStr=Inherit: Inherit via back propagation  ClampingZeroOutMin=[]  ClampingZeroOutMax=[]  FilterDenConstantOutDataTypeStr=Inherit: Inherit via back propagation  FilterDenConstantOutMin=[]  FilterDenConstantOutMax=[]  PCopyOutDataTypeStr=Inherit: Inherit via back propagation  PCopyOutMin=[]  PCopyOutMax=[]  NCopyOutDataTypeStr=Inherit: Inherit via back propagation  NCopyOutMin=[]  NCopyOutMax=[]  IntegratorContinuousStateAttributes=''  IntegratorStateMustResolveToSignalObject=off  IntegratorRTWStateStorageClass=Auto  FilterContinuousStateAttributes=''  FilterStateMustResolveToSignalObject=off  FilterRTWStateStorageClass=Auto  ParallelPVariant=InternalParameters  IdealPVariant=Disabled  IVariant=InternalParameters  DVariant=InternalParameters  IntegratorVariant=Discrete  SatVariant=Disabled  AWVariant=Passthrough  PCopyVariant=Disabled  TRVariant=Disabled  FdbkBlocksVariant=Forward  IdealPFdbkVariant=Disabled  SatFdbkVariant=Disabled  DerivativeFilterVariant=ForwardEulerFilter  NVariant=InternalParameters  NCopyVariant=Disabled  FilterICVariant=InternalICsFilter  IntegratorICVariant=InternalICs  ExternalResetVariant=Disabled  TRSumVariant=Passthrough  SumFdbkVariant=Disabled  SumVariant=Sum_PID  TsampFilterVariant=InternalTs  TsampNgainVariant=Passthrough  TsampIntegralVariant=Disabled_SignalSpec  ExternalSaturationOutDataTypeStr=Inherit: Same as second input  DerivativeSourceVariant=ErrorSignal  PreIntVariant=InternalPreInt
      settings: LibrarySourceBlock=simulink/Discrete/Discrete PID Controller
  Discrete PID Controller1 : slpidlib/PID Controller  Controller=PID  Form=Parallel  TimeDomain=Discrete-time  UseExternalTs=off  SampleTime=-1  IntegratorMethod=Forward Euler  FilterMethod=Forward Euler  ControllerParametersSource=internal  P=1  I=0  UseKiTs=off  D=0  UseExternalDerivativeSource=off  N=100  UseFilter=on  TunerSelectOption=Transfer Function Based (PID Tuner App)  InitialConditionSource=internal  InitialConditionForIntegrator=0  InitialConditionForFilter=0  DifferentiatorICPrevScaledInput=0  ExternalReset=none  TrackingMode=off  Kt=1  LimitOutput=off  SatLimitsSource=internal  UpperSaturationLimit=inf  LowerSaturationLimit=-inf  LinearizeAsGain=off  AntiWindupMode=none  Kb=1  LimitIntegrator=off  UpperIntegratorSaturationLimit=inf  LowerIntegratorSaturationLimit=-inf  POutMin=[]  POutMax=[]  IOutMin=[]  IOutMax=[]  DOutMin=[]  DOutMax=[]  NOutMin=[]  NOutMax=[]  SumOutMin=[]  SumOutMax=[]  SaturationOutMin=[]  SaturationOutMax=[]  PParamMin=[]  PParamMax=[]  IParamMin=[]  IParamMax=[]  DParamMin=[]  DParamMax=[]  NParamMin=[]  NParamMax=[]  KbParamMin=[]  KbParamMax=[]  KtParamMin=[]  KtParamMax=[]  KbOutMin=[]  KbOutMax=[]  KtOutMin=[]  KtOutMax=[]  IntegratorOutMin=[]  IntegratorOutMax=[]  FilterOutMin=[]  FilterOutMax=[]  SumI1OutMin=[]  SumI1OutMax=[]  SumI2OutMin=[]  SumI2OutMax=[]  SumI3OutMin=[]  SumI3OutMax=[]  SumI4OutMin=[]  SumI4OutMax=[]  SumDOutMin=[]  SumDOutMax=[]  DifferentiatorOutMin=[]  DifferentiatorOutMax=[]  FilterDiffOutCoefMin=[]  FilterDiffOutCoefMax=[]  ReciprocalOutMin=[]  ReciprocalOutMax=[]  SumDenOutMin=[]  SumDenOutMax=[]  SumNumOutMin=[]  SumNumOutMax=[]  DivideOutMin=[]  DivideOutMax=[]  UdiffTsProdOutMin=[]  UdiffTsProdOutMax=[]  NTsProdOutMin=[]  NTsProdOutMax=[]  UintegralTsProdOutMin=[]  UintegralTsProdOutMax=[]  UngainTsProdOutMin=[]  UngainTsProdOutMax=[]  ClampingZeroOutDataTypeStr=Inherit: Inherit via back propagation  ClampingZeroOutMin=[]  ClampingZeroOutMax=[]  FilterDenConstantOutDataTypeStr=Inherit: Inherit via back propagation  FilterDenConstantOutMin=[]  FilterDenConstantOutMax=[]  PCopyOutDataTypeStr=Inherit: Inherit via back propagation  PCopyOutMin=[]  PCopyOutMax=[]  NCopyOutDataTypeStr=Inherit: Inherit via back propagation  NCopyOutMin=[]  NCopyOutMax=[]  IntegratorContinuousStateAttributes=''  IntegratorStateMustResolveToSignalObject=off  IntegratorRTWStateStorageClass=Auto  FilterContinuousStateAttributes=''  FilterStateMustResolveToSignalObject=off  FilterRTWStateStorageClass=Auto  ParallelPVariant=InternalParameters  IdealPVariant=Disabled  IVariant=InternalParameters  DVariant=InternalParameters  IntegratorVariant=Discrete  SatVariant=Disabled  AWVariant=Passthrough  PCopyVariant=Disabled  TRVariant=Disabled  FdbkBlocksVariant=Forward  IdealPFdbkVariant=Disabled  SatFdbkVariant=Disabled  DerivativeFilterVariant=ForwardEulerFilter  NVariant=InternalParameters  NCopyVariant=Disabled  FilterICVariant=InternalICsFilter  IntegratorICVariant=InternalICs  ExternalResetVariant=Disabled  TRSumVariant=Passthrough  SumFdbkVariant=Disabled  SumVariant=Sum_PID  TsampFilterVariant=InternalTs  TsampNgainVariant=Passthrough  TsampIntegralVariant=Disabled_SignalSpec  ExternalSaturationOutDataTypeStr=Inherit: Same as second input  DerivativeSourceVariant=ErrorSignal  PreIntVariant=InternalPreInt
      settings: LibrarySourceBlock=simulink/Discrete/Discrete PID Controller
  Matrix Multiply : Product  Multiplication=Matrix(*)
  Mux2 : Mux  Inputs=3
  Mux3 : Mux  Inputs=3
  Rotation Angles to Direction Cosine Matrix : Angle2Dcm
      settings: AttributesFormatString=Rotation Order: %<rotationOrder>
  Selector : Selector  InputPortWidth=3  IndexOptions=Index vector (dialog)  Indices=[1]  OutputSizes=1
  Selector1 : Selector  InputPortWidth=3  IndexOptions=Index vector (dialog)  Indices=[2]  OutputSizes=1
  Sum : Sum  Inputs=|+-
  Sum1 : Sum  Inputs=|+-
  Out Bus Element : Outport  PortName=CmdHozirontalVelocity  Element=vXBody
  Out Bus Element1 : Outport  PortName=CmdHozirontalVelocity  Element=vYBody
  wires:
  Sum/1 -> Discrete PID Controller/1
  Mux2/1 -> Matrix Multiply/2
  Rotation Angles to Direction Cosine Matrix/1 -> Matrix Multiply/1
  Mux3/1 -> Rotation Angles to Direction Cosine Matrix/1
  Constant1/1 -> Mux3/2, Mux3/3
  Matrix Multiply/1 -> Selector1/1, Selector/1
  Selector/1 -> Out Bus Element/1
  Selector1/1 -> Out Bus Element1/1
  Cmd/1 -> Demux/1
  Sum1/1 -> Discrete PID Controller1/1
  Demux/1 -> [cmdx]
  [cmdx] -> Sum/1
  Demux/2 -> [cmdY]
  [cmdY] -> Sum1/1
  [y] -> Sum1/2
  [x] -> Sum/2
  Discrete PID Controller/1 -> [A1]
  [A1] -> Mux2/1
  Discrete PID Controller1/1 -> [A2]
  [A2] -> Mux2/2
  Constant/1 -> Mux2/3
  In Bus Element2/1 -> [x]
  In Bus Element1/1 -> [y]
  In Bus Element/1 -> [Yaw]
  [Yaw] -> Mux3/1

== system SimulinkOminidirectinalDrone_restored_from_autosave/Subsystem3/Horizontal Velocity Control ==
  In Bus Element1 : Inport  PortName=CmdHozirontalVelocity  Element=vYBody
  In Bus Element : Inport  PortName=CmdHozirontalVelocity  Element=vXBody
  In Bus Element2 : Inport  Port=2  PortName=Sensing  Element=vYBody
  In Bus Element3 : Inport  Port=2  PortName=Sensing  Element=vXBody
  Demux : Demux  Outputs=2
  Discrete PID Controller : slpidlib/PID Controller  Controller=PID  Form=Parallel  TimeDomain=Discrete-time  UseExternalTs=off  SampleTime=-1  IntegratorMethod=Forward Euler  FilterMethod=Forward Euler  ControllerParametersSource=internal  P=1  I=0  UseKiTs=off  D=0  UseExternalDerivativeSource=off  N=100  UseFilter=on  TunerSelectOption=Transfer Function Based (PID Tuner App)  InitialConditionSource=internal  InitialConditionForIntegrator=0  InitialConditionForFilter=0  DifferentiatorICPrevScaledInput=0  ExternalReset=none  TrackingMode=off  Kt=1  LimitOutput=off  SatLimitsSource=internal  UpperSaturationLimit=inf  LowerSaturationLimit=-inf  LinearizeAsGain=off  AntiWindupMode=none  Kb=1  LimitIntegrator=off  UpperIntegratorSaturationLimit=inf  LowerIntegratorSaturationLimit=-inf  POutMin=[]  POutMax=[]  IOutMin=[]  IOutMax=[]  DOutMin=[]  DOutMax=[]  NOutMin=[]  NOutMax=[]  SumOutMin=[]  SumOutMax=[]  SaturationOutMin=[]  SaturationOutMax=[]  PParamMin=[]  PParamMax=[]  IParamMin=[]  IParamMax=[]  DParamMin=[]  DParamMax=[]  NParamMin=[]  NParamMax=[]  KbParamMin=[]  KbParamMax=[]  KtParamMin=[]  KtParamMax=[]  KbOutMin=[]  KbOutMax=[]  KtOutMin=[]  KtOutMax=[]  IntegratorOutMin=[]  IntegratorOutMax=[]  FilterOutMin=[]  FilterOutMax=[]  SumI1OutMin=[]  SumI1OutMax=[]  SumI2OutMin=[]  SumI2OutMax=[]  SumI3OutMin=[]  SumI3OutMax=[]  SumI4OutMin=[]  SumI4OutMax=[]  SumDOutMin=[]  SumDOutMax=[]  DifferentiatorOutMin=[]  DifferentiatorOutMax=[]  FilterDiffOutCoefMin=[]  FilterDiffOutCoefMax=[]  ReciprocalOutMin=[]  ReciprocalOutMax=[]  SumDenOutMin=[]  SumDenOutMax=[]  SumNumOutMin=[]  SumNumOutMax=[]  DivideOutMin=[]  DivideOutMax=[]  UdiffTsProdOutMin=[]  UdiffTsProdOutMax=[]  NTsProdOutMin=[]  NTsProdOutMax=[]  UintegralTsProdOutMin=[]  UintegralTsProdOutMax=[]  UngainTsProdOutMin=[]  UngainTsProdOutMax=[]  ClampingZeroOutDataTypeStr=Inherit: Inherit via back propagation  ClampingZeroOutMin=[]  ClampingZeroOutMax=[]  FilterDenConstantOutDataTypeStr=Inherit: Inherit via back propagation  FilterDenConstantOutMin=[]  FilterDenConstantOutMax=[]  PCopyOutDataTypeStr=Inherit: Inherit via back propagation  PCopyOutMin=[]  PCopyOutMax=[]  NCopyOutDataTypeStr=Inherit: Inherit via back propagation  NCopyOutMin=[]  NCopyOutMax=[]  IntegratorContinuousStateAttributes=''  IntegratorStateMustResolveToSignalObject=off  IntegratorRTWStateStorageClass=Auto  FilterContinuousStateAttributes=''  FilterStateMustResolveToSignalObject=off  FilterRTWStateStorageClass=Auto  ParallelPVariant=InternalParameters  IdealPVariant=Disabled  IVariant=InternalParameters  DVariant=InternalParameters  IntegratorVariant=Discrete  SatVariant=Disabled  AWVariant=Passthrough  PCopyVariant=Disabled  TRVariant=Disabled  FdbkBlocksVariant=Forward  IdealPFdbkVariant=Disabled  SatFdbkVariant=Disabled  DerivativeFilterVariant=ForwardEulerFilter  NVariant=InternalParameters  NCopyVariant=Disabled  FilterICVariant=InternalICsFilter  IntegratorICVariant=InternalICs  ExternalResetVariant=Disabled  TRSumVariant=Passthrough  SumFdbkVariant=Disabled  SumVariant=Sum_PID  TsampFilterVariant=InternalTs  TsampNgainVariant=Passthrough  TsampIntegralVariant=Disabled_SignalSpec  ExternalSaturationOutDataTypeStr=Inherit: Same as second input  DerivativeSourceVariant=ErrorSignal  PreIntVariant=InternalPreInt
      settings: LibrarySourceBlock=simulink/Discrete/Discrete PID Controller
  Gain : Gain  Gain=-1
  Gain1 : Gain  Gain=1.1/g
  Mux : Mux  Inputs=2
  Mux1 : Mux  Inputs=2
  Mux2 : Mux  Inputs=2
  Selector : Selector  InputPortWidth=2  IndexOptions=Index vector (dialog)  Indices=[2]  OutputSizes=1
  Selector1 : Selector  InputPortWidth=2  IndexOptions=Index vector (dialog)  Indices=[1]  OutputSizes=1
  Sum : Sum  Inputs=|+-
  Tan : Trigonometry  Operator=tan
  Out Bus Element : Outport  PortName=CmdAttitude  Element=roll
  Out Bus Element1 : Outport  PortName=CmdAttitude  Element=pitch
  wires:
  In Bus Element/1 -> Mux/1
  In Bus Element1/1 -> Mux/2
  In Bus Element3/1 -> Mux1/1
  In Bus Element2/1 -> Mux1/2
  Mux/1 -> Sum/1
  Mux1/1 -> Sum/2
  Sum/1 -> Discrete PID Controller/1
  Discrete PID Controller/1 -> Selector/1, Selector1/1
  Selector1/1 -> Gain/1  "CmdAccXBody"
  Selector/1 -> Mux2/1  "CmdAccYBody"
  Gain/1 -> Mux2/2
  Mux2/1 -> Gain1/1
  Gain1/1 -> Tan/1
  Tan/1 -> Demux/1
  Demux/1 -> Out Bus Element/1
  Demux/2 -> Out Bus Element1/1

== system SimulinkOminidirectinalDrone_restored_from_autosave/Subsystem3/Subsystem ==
  Xe : Inport
  Euler : Inport  Port=2
  Ve : Inport  Port=3
  Demux : Demux  Outputs=3
  MATLAB Function : MATLAB Function  TreatAsAtomicUnit=on
  MATLAB Function1 : MATLAB Function  TreatAsAtomicUnit=on
  Rate Transition : RateTransition
  Rate Transition1 : RateTransition
  Subsystem : Subsystem
  wires:
  Euler/1 -> Rate Transition/1
  Ve/1 -> Rate Transition1/1
  Xe/1 -> Demux/1
  Demux/1 -> MATLAB Function1/1(Xe)
  Demux/2 -> MATLAB Function1/2(Ye)

== system SimulinkOminidirectinalDrone_restored_from_autosave/Subsystem3/Subsystem1 ==
  In1 : Inport
  Constant : Constant  Commented=on  Value=[0 0 0]
  Constant1 : Constant  Commented=on
  Constant2 : Constant  Commented=on  Value=[0 0 0;5 0 0;5 5 0 ; 0 5 0; 0 0 0]
  Constant3 : Constant  Commented=on  Value=0.2
  Integrator : Integrator  Commented=on
  Ramp : simulink/Sources/Ramp  Commented=on  slope=10  start=0  InitialOutput=0
  Selector : Selector  Commented=on  InputPortWidth=3  IndexOptions=Index vector (dialog)  Indices=[1 2]  OutputSizes=1
  Selector1 : Selector  Commented=on  InputPortWidth=3  IndexOptions=Index vector (dialog)  Indices=[3]  OutputSizes=1
  Switch : Switch  Commented=on  Criteria=u2 > Threshold  Threshold=5  SaturateOnIntegerOverflow=off  InputSameDT=off
  Terminator2 : Terminator  Commented=on
  Terminator3 : Terminator  Commented=on
  Vector Concatenate : Concatenate  Commented=on
  Waypoint Follower : uavalgslib/Waypoint Follower  Commented=on  UAVType=multirotor  StartFrom=first  TransitionRadiusSource=internal  TransitionRadius=10  MinLookaheadDistance=0.1  HoverAtLastWaypoint=off  YawInput=off  ShowCrossTrackErrorOutput=off  ShowStatusOutput=off  SimulateUsing=Interpreted execution
  Out1 : Outport
  Out4 : Outport  Port=2
  Out2 : Outport  Port=3
  Out3 : Outport  Port=4
  wires:
  Waypoint Follower/1 -> Selector/1, Selector1/1
  Integrator/1 -> Switch/1
  Ramp/1 -> Switch/2
  Switch/1 -> Vector Concatenate/1
  Selector/1 -> Out1/1
  Selector1/1 -> Out3/1
  Vector Concatenate/1 -> Waypoint Follower/1
  Constant/1 -> Switch/3
  Constant3/1 -> Waypoint Follower/3
  Constant1/1 -> Vector Concatenate/2
  Constant2/1 -> Waypoint Follower/2
  Waypoint Follower/4 -> Terminator3/1
  Waypoint Follower/2 -> Terminator2/1
  In1/1 -> Integrator/1
  Waypoint Follower/3 -> Out2/1
